simulink library "mylib"  (R2020a)
settings: Solver=VariableStepAuto  StartTime=0.0  StopTime=10.0  RelTol=1e-3
undefined symbols (not defined in the file): d_du_max_pu, dir_to_bus1, dir_to_bus_0L, dir_to_bus_2, dir_to_line1, dir_to_line_0L, dir_to_line_2, du_max_pu, du_ph_max_pu, Fi_0, Fi_T_H, Fi_T_L, Fi_T_M, I0_calc_0L, I0_comp_H, I0_comp_L, I0_comp_M, I0_max_0L, I2_max_2, I_diff1, I_diff2, I_diff3, I_diff4, I_diff5, I_diff_to, I_hight_CT1_G, I_hight_CT2_G, I_low_CT1, I_low_CT2, I_max1, I_max2, I_max3, I_max4, I_max5, I_min_sec_CT1, I_min_sec_CT2, I_unb, Iph_max_0L, Iph_max_2, jmp_in_zone, jmp_in_zone_0L, jmp_in_zone_2, K_dop, max_min1, only_K1_0L, only_K1_2, only_K2_0L, only_K2_2, only_K3_0L, only_K3_2, P_ctl_0, PQ_Fi_ctl_0, Q_ctl_0, S_set_0, set, set1, T_fast, T_I_ctl, T_off, T_on ... (+15)
libraries: $bdroot x184, powerlib_meascontrol x97
(part 7 of 14)

== system mylib/278_dzt_v1/diff_brake/calc_brake_Ia ==
  I_max : Inport
  I_diff_to : Inport  Port=2
  I_diff_1 : Inport  Port=3
  I_max_1 : Inport  Port=4
  I_diff_2 : Inport  Port=5
  I_max_2 : Inport  Port=6
  I_diff_3 : Inport  Port=7
  I_max_3 : Inport  Port=8
  I_diff_4 : Inport  Port=9
  I_max_4 : Inport  Port=10
  I_diff_5 : Inport  Port=11
  I_max_5 : Inport  Port=12
  31 : Constant  Value=0
  cut_brake_1 : Subsystem
  cut_brake_2 : Subsystem
  cut_brake_3 : Subsystem
  cut_brake_4 : Subsystem
  I_brake : Outport
  wires:
  I_diff_5/1 -> cut_brake_3/7(I_diff_next), cut_brake_4/5(I_diff_cur2)
  I_max_5/1 -> cut_brake_3/8(I_max_next), cut_brake_4/6(I_max_cur2)
  cut_brake_3/1(I_brake) -> cut_brake_4/1(Y_in)
  cut_brake_2/1(I_brake) -> cut_brake_3/1(Y_in)
  I_max_4/1 -> cut_brake_3/6(I_max_cur2), cut_brake_4/4(I_max_cur1), cut_brake_2/8(I_max_next)
  I_diff_4/1 -> cut_brake_2/7(I_diff_next), cut_brake_4/3(I_diff_cur1), cut_brake_3/5(I_diff_cur2)
  cut_brake_1/1(I_brake) -> cut_brake_2/1(Y_in)
  31/1 -> cut_brake_1/1(Y_in), cut_brake_4/7(I_diff_next), cut_brake_4/8(I_max_next)
  I_max/1 -> cut_brake_1/2(I_max), cut_brake_2/2(I_max), cut_brake_3/2(I_max), cut_brake_4/2(I_max)
  I_max_3/1 -> cut_brake_1/8(I_max_next), cut_brake_2/6(I_max_cur2), cut_brake_3/4(I_max_cur1)
  I_diff_3/1 -> cut_brake_1/7(I_diff_next), cut_brake_2/5(I_diff_cur2), cut_brake_3/3(I_diff_cur1)
  I_max_2/1 -> cut_brake_1/6(I_max_cur2), cut_brake_2/4(I_max_cur1)
  I_diff_2/1 -> cut_brake_1/5(I_diff_cur2), cut_brake_2/3(I_diff_cur1)
  I_max_1/1 -> cut_brake_1/4(I_max_cur1)
  I_diff_1/1 -> cut_brake_1/3(I_diff_cur1)
  I_diff_to/1 -> cut_brake_1/9(I_diff_to), cut_brake_2/9(I_diff_to), cut_brake_3/9(I_diff_to), cut_brake_4/9(I_diff_to)
  cut_brake_4/1(I_brake) -> I_brake/1

== system mylib/278_dzt_v1/diff_brake/calc_brake_Ib ==
  I_max : Inport
  I_diff_to : Inport  Port=2
  I_diff_1 : Inport  Port=3
  I_max_1 : Inport  Port=4
  I_diff_2 : Inport  Port=5
  I_max_2 : Inport  Port=6
  I_diff_3 : Inport  Port=7
  I_max_3 : Inport  Port=8
  I_diff_4 : Inport  Port=9
  I_max_4 : Inport  Port=10
  I_diff_5 : Inport  Port=11
  I_max_5 : Inport  Port=12
  31 : Constant  Value=0
  cut_brake_1 : Subsystem
  cut_brake_2 : Subsystem
  cut_brake_3 : Subsystem
  cut_brake_4 : Subsystem
  I_brake : Outport
  wires:
  I_diff_5/1 -> cut_brake_3/7(I_diff_next), cut_brake_4/5(I_diff_cur2)
  I_max_5/1 -> cut_brake_3/8(I_max_next), cut_brake_4/6(I_max_cur2)
  cut_brake_3/1(I_brake) -> cut_brake_4/1(Y_in)
  cut_brake_2/1(I_brake) -> cut_brake_3/1(Y_in)
  I_max_4/1 -> cut_brake_3/6(I_max_cur2), cut_brake_4/4(I_max_cur1), cut_brake_2/8(I_max_next)
  I_diff_4/1 -> cut_brake_2/7(I_diff_next), cut_brake_4/3(I_diff_cur1), cut_brake_3/5(I_diff_cur2)
  cut_brake_1/1(I_brake) -> cut_brake_2/1(Y_in)
  31/1 -> cut_brake_1/1(Y_in), cut_brake_4/7(I_diff_next), cut_brake_4/8(I_max_next)
  I_max/1 -> cut_brake_1/2(I_max), cut_brake_2/2(I_max), cut_brake_3/2(I_max), cut_brake_4/2(I_max)
  I_max_3/1 -> cut_brake_1/8(I_max_next), cut_brake_2/6(I_max_cur2), cut_brake_3/4(I_max_cur1)
  I_diff_3/1 -> cut_brake_1/7(I_diff_next), cut_brake_2/5(I_diff_cur2), cut_brake_3/3(I_diff_cur1)
  I_max_2/1 -> cut_brake_1/6(I_max_cur2), cut_brake_2/4(I_max_cur1)
  I_diff_2/1 -> cut_brake_1/5(I_diff_cur2), cut_brake_2/3(I_diff_cur1)
  I_max_1/1 -> cut_brake_1/4(I_max_cur1)
  I_diff_1/1 -> cut_brake_1/3(I_diff_cur1)
  I_diff_to/1 -> cut_brake_1/9(I_diff_to), cut_brake_2/9(I_diff_to), cut_brake_3/9(I_diff_to), cut_brake_4/9(I_diff_to)
  cut_brake_4/1(I_brake) -> I_brake/1

== system mylib/278_dzt_v1/diff_brake/calc_brake_Ic ==
  I_max : Inport
  I_diff_to : Inport  Port=2
  I_diff_1 : Inport  Port=3
  I_max_1 : Inport  Port=4
  I_diff_2 : Inport  Port=5
  I_max_2 : Inport  Port=6
  I_diff_3 : Inport  Port=7
  I_max_3 : Inport  Port=8
  I_diff_4 : Inport  Port=9
  I_max_4 : Inport  Port=10
  I_diff_5 : Inport  Port=11
  I_max_5 : Inport  Port=12
  31 : Constant  Value=0
  cut_brake_1 : Subsystem
  cut_brake_2 : Subsystem
  cut_brake_3 : Subsystem
  cut_brake_4 : Subsystem
  I_brake : Outport
  wires:
  I_diff_5/1 -> cut_brake_3/7(I_diff_next), cut_brake_4/5(I_diff_cur2)
  I_max_5/1 -> cut_brake_3/8(I_max_next), cut_brake_4/6(I_max_cur2)
  cut_brake_3/1(I_brake) -> cut_brake_4/1(Y_in)
  cut_brake_2/1(I_brake) -> cut_brake_3/1(Y_in)
  I_max_4/1 -> cut_brake_3/6(I_max_cur2), cut_brake_4/4(I_max_cur1), cut_brake_2/8(I_max_next)
  I_diff_4/1 -> cut_brake_2/7(I_diff_next), cut_brake_4/3(I_diff_cur1), cut_brake_3/5(I_diff_cur2)
  cut_brake_1/1(I_brake) -> cut_brake_2/1(Y_in)
  31/1 -> cut_brake_1/1(Y_in), cut_brake_4/7(I_diff_next), cut_brake_4/8(I_max_next)
  I_max/1 -> cut_brake_1/2(I_max), cut_brake_2/2(I_max), cut_brake_3/2(I_max), cut_brake_4/2(I_max)
  I_max_3/1 -> cut_brake_1/8(I_max_next), cut_brake_2/6(I_max_cur2), cut_brake_3/4(I_max_cur1)
  I_diff_3/1 -> cut_brake_1/7(I_diff_next), cut_brake_2/5(I_diff_cur2), cut_brake_3/3(I_diff_cur1)
  I_max_2/1 -> cut_brake_1/6(I_max_cur2), cut_brake_2/4(I_max_cur1)
  I_diff_2/1 -> cut_brake_1/5(I_diff_cur2), cut_brake_2/3(I_diff_cur1)
  I_max_1/1 -> cut_brake_1/4(I_max_cur1)
  I_diff_1/1 -> cut_brake_1/3(I_diff_cur1)
  I_diff_to/1 -> cut_brake_1/9(I_diff_to), cut_brake_2/9(I_diff_to), cut_brake_3/9(I_diff_to), cut_brake_4/9(I_diff_to)
  cut_brake_4/1(I_brake) -> I_brake/1

== system mylib/278_dzt_v1/diff_comp18_ph/diff_comp_a ==
  I_diff : Inport
  I_brake : Inport  Port=2
  I_diff_to : Inport  Port=3
  10 : Logic  AllPortsSameDT=off  OutDataTypeStr=boolean
  11 : Logic  Operator=NOT  AllPortsSameDT=off  OutDataTypeStr=boolean
  2 : RelationalOperator  Operator=>  OutDataTypeStr=boolean  RndMeth=Simplest
  25 : Constant  Value=0
  3 : RelationalOperator  Operator=>  OutDataTypeStr=boolean  RndMeth=Simplest
  4 : RelationalOperator  Operator===  OutDataTypeStr=boolean  RndMeth=Simplest
  5 : RelationalOperator  Operator===  OutDataTypeStr=boolean  RndMeth=Simplest
  7 : Logic  Operator=OR  AllPortsSameDT=off  OutDataTypeStr=boolean
  8 : Logic  AllPortsSameDT=off  OutDataTypeStr=boolean
  9 : Logic  Operator=NOT  AllPortsSameDT=off  OutDataTypeStr=boolean
  Y : Outport
  wires:
  7/1 -> Y/1
  10/1 -> 7/2
  8/1 -> 7/1
  5/1 -> 11/1
  4/1 -> 9/1
  3/1 -> 10/1
  2/1 -> 8/1
  9/1 -> 8/2
  11/1 -> 10/2
  25/1 -> 5/2, 4/2
  I_diff_to/1 -> 3/2, 5/1
  I_brake/1 -> 2/2, 4/1
  I_diff/1 -> 2/1, 3/1

== system mylib/278_dzt_v1/diff_comp18_ph/diff_comp_b ==
  I_diff : Inport
  I_brake : Inport  Port=2
  I_diff_to : Inport  Port=3
  10 : Logic  AllPortsSameDT=off  OutDataTypeStr=boolean
  11 : Logic  Operator=NOT  AllPortsSameDT=off  OutDataTypeStr=boolean
  2 : RelationalOperator  Operator=>  OutDataTypeStr=boolean  RndMeth=Simplest
  25 : Constant  Value=0
  3 : RelationalOperator  Operator=>  OutDataTypeStr=boolean  RndMeth=Simplest
  4 : RelationalOperator  Operator===  OutDataTypeStr=boolean  RndMeth=Simplest
  5 : RelationalOperator  Operator===  OutDataTypeStr=boolean  RndMeth=Simplest
  7 : Logic  Operator=OR  AllPortsSameDT=off  OutDataTypeStr=boolean
  8 : Logic  AllPortsSameDT=off  OutDataTypeStr=boolean
  9 : Logic  Operator=NOT  AllPortsSameDT=off  OutDataTypeStr=boolean
  Y : Outport
  wires:
  7/1 -> Y/1
  10/1 -> 7/2
  8/1 -> 7/1
  5/1 -> 11/1
  4/1 -> 9/1
  3/1 -> 10/1
  2/1 -> 8/1
  9/1 -> 8/2
  11/1 -> 10/2
  25/1 -> 5/2, 4/2
  I_diff_to/1 -> 3/2, 5/1
  I_brake/1 -> 2/2, 4/1
  I_diff/1 -> 2/1, 3/1

== system mylib/278_dzt_v1/diff_comp18_ph/diff_comp_c ==
  I_diff : Inport
  I_brake : Inport  Port=2
  I_diff_to : Inport  Port=3
  10 : Logic  AllPortsSameDT=off  OutDataTypeStr=boolean
  11 : Logic  Operator=NOT  AllPortsSameDT=off  OutDataTypeStr=boolean
  2 : RelationalOperator  Operator=>  OutDataTypeStr=boolean  RndMeth=Simplest
  25 : Constant  Value=0
  3 : RelationalOperator  Operator=>  OutDataTypeStr=boolean  RndMeth=Simplest
  4 : RelationalOperator  Operator===  OutDataTypeStr=boolean  RndMeth=Simplest
  5 : RelationalOperator  Operator===  OutDataTypeStr=boolean  RndMeth=Simplest
  7 : Logic  Operator=OR  AllPortsSameDT=off  OutDataTypeStr=boolean
  8 : Logic  AllPortsSameDT=off  OutDataTypeStr=boolean
  9 : Logic  Operator=NOT  AllPortsSameDT=off  OutDataTypeStr=boolean
  Y : Outport
  wires:
  7/1 -> Y/1
  10/1 -> 7/2
  8/1 -> 7/1
  5/1 -> 11/1
  4/1 -> 9/1
  3/1 -> 10/1
  2/1 -> 8/1
  9/1 -> 8/2
  11/1 -> 10/2
  25/1 -> 5/2, 4/2
  I_diff_to/1 -> 3/2, 5/1
  I_brake/1 -> 2/2, 4/1
  I_diff/1 -> 2/1, 3/1

== system mylib/278_dzt_v1/diff_trans_calc_H/Ia_calc ==
  I_re_in : Inport
  I_im_in : Inport  Port=2
  I30_re : Inport  Port=3
  I30_im : Inport  Port=4
  K_CT : Inport  Port=5
  K_T : Inport  Port=6
  I0_comp : Inport  Port=7
  Fi_CT : Inport  Port=8
  Fi_T : Inport  Port=9
  1 : Constant  Value=0.017453292519
  10 : Sum  Inputs=+-
  {2..4,11..13} (6 alike) : Product
  14 : Sum  Inputs=+-
  5 : Sum  Inputs=+-
  6 : Switch  Criteria=u2 > Threshold
  7 : Switch  Criteria=u2 > Threshold
  8 : Trigonometry
  9 : Trigonometry  Operator=cos
  module : $bdroot/module  SystemSampleTime=-1  Latency=0  AutoFrameSizeCalculation=off
  orto_MUL_orto : Subsystem
  orto_to_arg : Subsystem
  I_re : Outport
  I_im : Outport  Port=2
  I_eff : Outport  Port=3
  I_arg : Outport  Port=4
  wires:
  I0_comp/1 -> 7/2, 6/2
  14/1 -> 6/1
  5/1 -> 7/1
  13/1 -> 14/2
  12/1 -> 5/2
  4/1 -> 14/1, 6/3
  3/1 -> 5/1, 7/3
  2/1 -> 3/2, 4/2, 12/2, 13/2
  I30_im/1 -> 13/1
  I30_re/1 -> 12/1
  11/1 -> 9/1, 8/1
  1/1 -> 11/2
  10/1 -> 11/1
  Fi_T/1 -> 10/2
  Fi_CT/1 -> 10/1
  8/1 -> orto_MUL_orto/4(F2im)
  9/1 -> orto_MUL_orto/3(F2re)
  7/1 -> orto_MUL_orto/1(F1re)
  6/1 -> orto_MUL_orto/2(F1im)
  orto_MUL_orto/2(Fim) -> I_im/1, module/2, orto_to_arg/2(im)
  orto_MUL_orto/1(Fre) -> I_re/1, module/1, orto_to_arg/1(re)
  module/1 -> I_eff/1
  orto_to_arg/1(arg) -> I_arg/1
  I_im_in/1 -> 4/1
  I_re_in/1 -> 3/1
  K_T/1 -> 2/2
  K_CT/1 -> 2/1

== system mylib/278_dzt_v1/diff_trans_calc_H/Ia_diff_calc ==
  I_re_1 : Inport
  I_im_1 : Inport  Port=2
  I_re_2 : Inport  Port=3
  I_im_2 : Inport  Port=4
  fix : Inport  Port=5
  I_re_max_in : Inport  Port=6
  I_im_max_in : Inport  Port=7
  in_range_I : Inport  Port=8
  {1,3..6,12} (6 alike) : Switch  Criteria=u2 > Threshold
  10 : RelationalOperator  Operator=>  OutDataTypeStr=boolean  RndMeth=Simplest
  11 : Sum
  154 : Constant  Value=0
  2 : Sum
  module1 : Subsystem
  module2 : Subsystem
  I_re_diff : Outport
  I_im_diff1 : Outport  Port=2
  I_re_max : Outport  Port=3
  I_im_max : Outport  Port=4
  wires:
  fix/1 -> 4/2, 3/2
  I_re_2/1 -> 6/3
  I_im_2/1 -> 5/3
  I_im_max_in/1 -> module1/2(Im), 1/1
  I_re_max_in/1 -> 12/1, module1/1(Re)
  4/1 -> 2/2, 12/3, module2/1(Re)
  3/1 -> 1/3, 11/2, module2/2(Im)
  154/1 -> 5/1, 6/1, 4/3, 3/3
  in_range_I/1 -> 5/2, 6/2
  5/1 -> 3/1
  6/1 -> 4/1
  module2/1(Module) -> 10/2
  module1/1(Module) -> 10/1
  I_im_1/1 -> 11/1
  I_re_1/1 -> 2/1
  10/1 -> 1/2, 12/2
  2/1 -> I_re_diff/1
  11/1 -> I_im_diff1/1
  1/1 -> I_im_max/1
  12/1 -> I_re_max/1

== system mylib/278_dzt_v1/diff_trans_calc_H/Ib_calc ==
  I_re_in : Inport
  I_im_in : Inport  Port=2
  I30_re : Inport  Port=3
  I30_im : Inport  Port=4
  K_CT : Inport  Port=5
  K_T : Inport  Port=6
  I0_comp : Inport  Port=7
  Fi_CT : Inport  Port=8
  Fi_T : Inport  Port=9
  1 : Constant  Value=0.017453292519
  10 : Sum  Inputs=+-
  {2..4,11..13} (6 alike) : Product
  14 : Sum  Inputs=+-
  5 : Sum  Inputs=+-
  6 : Switch  Criteria=u2 > Threshold
  7 : Switch  Criteria=u2 > Threshold
  8 : Trigonometry
  9 : Trigonometry  Operator=cos
  module : $bdroot/module  SystemSampleTime=-1  Latency=0  AutoFrameSizeCalculation=off
  orto_MUL_orto : Subsystem
  orto_to_arg : Subsystem
  I_re : Outport
  I_im : Outport  Port=2
  I_eff : Outport  Port=3
  I_arg : Outport  Port=4
  wires:
  I0_comp/1 -> 7/2, 6/2
  14/1 -> 6/1
  5/1 -> 7/1
  13/1 -> 14/2
  12/1 -> 5/2
  4/1 -> 14/1, 6/3
  3/1 -> 5/1, 7/3
  2/1 -> 3/2, 4/2, 12/2, 13/2
  I30_im/1 -> 13/1
  I30_re/1 -> 12/1
  11/1 -> 9/1, 8/1
  1/1 -> 11/2
  10/1 -> 11/1
  Fi_T/1 -> 10/2
  Fi_CT/1 -> 10/1
  8/1 -> orto_MUL_orto/4(F2im)
  9/1 -> orto_MUL_orto/3(F2re)
  7/1 -> orto_MUL_orto/1(F1re)
  6/1 -> orto_MUL_orto/2(F1im)
  orto_MUL_orto/2(Fim) -> I_im/1, module/2, orto_to_arg/2(im)
  orto_MUL_orto/1(Fre) -> I_re/1, module/1, orto_to_arg/1(re)
  module/1 -> I_eff/1
  orto_to_arg/1(arg) -> I_arg/1
  I_im_in/1 -> 4/1
  I_re_in/1 -> 3/1
  K_T/1 -> 2/2
  K_CT/1 -> 2/1

== system mylib/278_dzt_v1/diff_trans_calc_H/Ib_diff_calc ==
  I_re_1 : Inport
  I_im_1 : Inport  Port=2
  I_re_2 : Inport  Port=3
  I_im_2 : Inport  Port=4
  fix : Inport  Port=5
  I_re_max_in : Inport  Port=6
  I_im_max_in : Inport  Port=7
  in_range_I : Inport  Port=8
  {1,3..6,12} (6 alike) : Switch  Criteria=u2 > Threshold
  10 : RelationalOperator  Operator=>  OutDataTypeStr=boolean  RndMeth=Simplest
  11 : Sum
  154 : Constant  Value=0
  2 : Sum
  module1 : Subsystem
  module2 : Subsystem
  I_re_diff : Outport
  I_im_diff1 : Outport  Port=2
  I_re_max : Outport  Port=3
  I_im_max : Outport  Port=4
  wires:
  fix/1 -> 4/2, 3/2
  I_re_2/1 -> 6/3
  I_im_2/1 -> 5/3
  I_im_max_in/1 -> module1/2(Im), 1/1
  I_re_max_in/1 -> 12/1, module1/1(Re)
  4/1 -> 2/2, 12/3, module2/1(Re)
  3/1 -> 1/3, 11/2, module2/2(Im)
  154/1 -> 5/1, 6/1, 4/3, 3/3
  in_range_I/1 -> 5/2, 6/2
  5/1 -> 3/1
  6/1 -> 4/1
  module2/1(Module) -> 10/2
  module1/1(Module) -> 10/1
  I_im_1/1 -> 11/1
  I_re_1/1 -> 2/1
  10/1 -> 1/2, 12/2
  2/1 -> I_re_diff/1
  11/1 -> I_im_diff1/1
  1/1 -> I_im_max/1
  12/1 -> I_re_max/1

== system mylib/278_dzt_v1/diff_trans_calc_H/Ic_calc ==
  I_re_in : Inport
  I_im_in : Inport  Port=2
  I30_re : Inport  Port=3
  I30_im : Inport  Port=4
  K_CT : Inport  Port=5
  K_T : Inport  Port=6
  I0_comp : Inport  Port=7
  Fi_CT : Inport  Port=8
  Fi_T : Inport  Port=9
  1 : Constant  Value=0.017453292519
  10 : Sum  Inputs=+-
  {2..4,11..13} (6 alike) : Product
  14 : Sum  Inputs=+-
  5 : Sum  Inputs=+-
  6 : Switch  Criteria=u2 > Threshold
  7 : Switch  Criteria=u2 > Threshold
  8 : Trigonometry
  9 : Trigonometry  Operator=cos
  module : $bdroot/module  SystemSampleTime=-1  Latency=0  AutoFrameSizeCalculation=off
  orto_MUL_orto : Subsystem
  orto_to_arg : Subsystem
  I_re : Outport
  I_im : Outport  Port=2
  I_eff : Outport  Port=3
  I_arg : Outport  Port=4
  wires:
  I0_comp/1 -> 7/2, 6/2
  14/1 -> 6/1
  5/1 -> 7/1
  13/1 -> 14/2
  12/1 -> 5/2
  4/1 -> 14/1, 6/3
  3/1 -> 5/1, 7/3
  2/1 -> 3/2, 4/2, 12/2, 13/2
  I30_im/1 -> 13/1
  I30_re/1 -> 12/1
  11/1 -> 9/1, 8/1
  1/1 -> 11/2
  10/1 -> 11/1
  Fi_T/1 -> 10/2
  Fi_CT/1 -> 10/1
  8/1 -> orto_MUL_orto/4(F2im)
  9/1 -> orto_MUL_orto/3(F2re)
  7/1 -> orto_MUL_orto/1(F1re)
  6/1 -> orto_MUL_orto/2(F1im)
  orto_MUL_orto/2(Fim) -> I_im/1, module/2, orto_to_arg/2(im)
  orto_MUL_orto/1(Fre) -> I_re/1, module/1, orto_to_arg/1(re)
  module/1 -> I_eff/1
  orto_to_arg/1(arg) -> I_arg/1
  I_im_in/1 -> 4/1
  I_re_in/1 -> 3/1
  K_T/1 -> 2/2
  K_CT/1 -> 2/1

== system mylib/278_dzt_v1/diff_trans_calc_H/Ic_diff_calc ==
  I_re_1 : Inport
  I_im_1 : Inport  Port=2
  I_re_2 : Inport  Port=3
  I_im_2 : Inport  Port=4
  fix : Inport  Port=5
  I_re_max_in : Inport  Port=6
  I_im_max_in : Inport  Port=7
  in_range_I : Inport  Port=8
  {1,3..6,12} (6 alike) : Switch  Criteria=u2 > Threshold
  10 : RelationalOperator  Operator=>  OutDataTypeStr=boolean  RndMeth=Simplest
  11 : Sum
  154 : Constant  Value=0
  2 : Sum
  module1 : Subsystem
  module2 : Subsystem
  I_re_diff : Outport
  I_im_diff1 : Outport  Port=2
  I_re_max : Outport  Port=3
  I_im_max : Outport  Port=4
  wires:
  fix/1 -> 4/2, 3/2
  I_re_2/1 -> 6/3
  I_im_2/1 -> 5/3
  I_im_max_in/1 -> module1/2(Im), 1/1
  I_re_max_in/1 -> 12/1, module1/1(Re)
  4/1 -> 2/2, 12/3, module2/1(Re)
  3/1 -> 1/3, 11/2, module2/2(Im)
  154/1 -> 5/1, 6/1, 4/3, 3/3
  in_range_I/1 -> 5/2, 6/2
  5/1 -> 3/1
  6/1 -> 4/1
  module2/1(Module) -> 10/2
  module1/1(Module) -> 10/1
  I_im_1/1 -> 11/1
  I_re_1/1 -> 2/1
  10/1 -> 1/2, 12/2
  2/1 -> I_re_diff/1
  11/1 -> I_im_diff1/1
  1/1 -> I_im_max/1
  12/1 -> I_re_max/1

== system mylib/278_dzt_v1/diff_trans_calc_H/jmp_cnt18_ph ==
  cnt_jmp0_in : Inport
  cnt_jmp_in : Inport  Port=2
  Ia_zero_in : Inport  Port=3
  Ib_zero_in : Inport  Port=4
  Ic_zero_in : Inport  Port=5
  Iall_zero_in : Inport  Port=6
  in_range_Ia : Inport  Port=7
  in_range_Ib : Inport  Port=8
  in_range_Ic : Inport  Port=9
  jmp_Ia : Inport  Port=10
  jmp_Ib : Inport  Port=11
  jmp_Ic : Inport  Port=12
  fix : Inport  Port=13
  {1,3,5..7,10} (6 alike) : Logic  AllPortsSameDT=off  OutDataTypeStr=boolean
  11 : Logic  Operator=NOT  AllPortsSameDT=off  OutDataTypeStr=boolean
  12 : Logic  Operator=OR  AllPortsSameDT=off  OutDataTypeStr=boolean
  13 : Logic  Operator=OR  AllPortsSameDT=off  OutDataTypeStr=boolean
  14 : Logic  Operator=OR  AllPortsSameDT=off  OutDataTypeStr=boolean
  15 : Logic  Inputs=4  AllPortsSameDT=off  OutDataTypeStr=boolean
  16 : Switch  Criteria=u2 > Threshold
  17 : Switch  Criteria=u2 > Threshold
  18 : Sum
  19 : Constant
  2 : Logic  Operator=NOT  AllPortsSameDT=off  OutDataTypeStr=boolean
  20 : Sum
  21 : Constant
  4 : Logic  Operator=NOT  AllPortsSameDT=off  OutDataTypeStr=boolean
  8 : Logic  Operator=OR  Inputs=3  AllPortsSameDT=off  OutDataTypeStr=boolean
  9 : Logic  Operator=OR  Inputs=3  AllPortsSameDT=off  OutDataTypeStr=boolean
  R_TRIG : $bdroot/R_TRIG  SystemSampleTime=-1  Latency=0  AutoFrameSizeCalculation=off
  R_TRIG1 : $bdroot/R_TRIG  SystemSampleTime=-1  Latency=0  AutoFrameSizeCalculation=off
  R_TRIG2 : $bdroot/R_TRIG  SystemSampleTime=-1  Latency=0  AutoFrameSizeCalculation=off
  cnt_jmp0 : Outport
  cnt_jmp : Outport  Port=2
  Ia_zero : Outport  Port=3
  Ib_zero : Outport  Port=4
  Ic_zero : Outport  Port=5
  Iall_zero : Outport  Port=6
  wires:
  cnt_jmp0_in/1 -> 16/3, 20/1
  R_TRIG2/1 -> 9/3, 6/2
  fix/1 -> 10/2, 1/2, 3/2
  cnt_jmp_in/1 -> 17/3, 18/1
  9/1 -> 17/2
  20/1 -> 16/1
  21/1 -> 20/2
  19/1 -> 18/2
  18/1 -> 17/1
  17/1 -> cnt_jmp/1
  16/1 -> cnt_jmp0/1
  8/1 -> 16/2
  15/1 -> Iall_zero/1
  14/1 -> Ic_zero/1
  13/1 -> Ib_zero/1
  12/1 -> Ia_zero/1
  Ia_zero_in/1 -> 12/1
  Ib_zero_in/1 -> 13/1
  Ic_zero_in/1 -> 14/1
  Iall_zero_in/1 -> 15/1
  R_TRIG1/1 -> 9/2, 5/2
  R_TRIG/1 -> 9/1, 7/2
  6/1 -> 8/3
  7/1 -> 8/1
  5/1 -> 8/2
  10/1 -> 6/1, 15/4, 14/2
  1/1 -> 5/1, 15/3, 13/2
  3/1 -> 7/1, 15/2, 12/2
  in_range_Ia/1 -> 4/1
  4/1 -> 3/1
  in_range_Ib/1 -> 2/1
  2/1 -> 1/1
  in_range_Ic/1 -> 11/1
  11/1 -> 10/1
  jmp_Ib/1 -> R_TRIG1/1
  jmp_Ic/1 -> R_TRIG2/1
  jmp_Ia/1 -> R_TRIG/1

== system mylib/278_dzt_v1/diff_trans_calc_H/simpcomp ==
  FAre : Inport
  FAim : Inport  Port=2
  FBre : Inport  Port=3
  FBim : Inport  Port=4
  FCre : Inport  Port=5
  FCim : Inport  Port=6
  1 : Constant  Value=-0.5
  {3..5,9..11,18..23} (12 alike) : Sum
  {2,12..16} (6 alike) : Product
  17 : Constant  Value=0.33333333333
  6 : Constant  Value=0.8660254037844386
  7 : Constant  Value=-0.8660254037844386
  orto_MUL_orto : Subsystem
  orto_MUL_orto1 : Subsystem
  orto_MUL_orto2 : Subsystem
  orto_MUL_orto3 : Subsystem
  F0re : Outport
  F0im : Outport  Port=2
  F1re : Outport  Port=3
  F1im : Outport  Port=4
  F2re : Outport  Port=5
  F2im : Outport  Port=6
  wires:
  1/1 -> orto_MUL_orto1/3(F2re), orto_MUL_orto/3(F2re), orto_MUL_orto2/3(F2re), orto_MUL_orto3/3(F2re)
  6/1 -> orto_MUL_orto2/4(F2im), orto_MUL_orto/4(F2im)
  7/1 -> orto_MUL_orto3/4(F2im), orto_MUL_orto1/4(F2im)
  15/1 -> F2im/1
  14/1 -> F2re/1
  16/1 -> F1im/1
  13/1 -> F1re/1
  2/1 -> F0re/1
  12/1 -> F0im/1
  5/1 -> 2/1
  3/1 -> 12/1
  4/1 -> 13/1
  11/1 -> 16/1
  9/1 -> 14/1
  10/1 -> 15/1
  20/1 -> 10/2
  23/1 -> 9/2
  21/1 -> 11/2
  22/1 -> 4/2
  18/1 -> 3/1
  19/1 -> 5/1
  FAim/1 -> 10/1, 3/2, 11/1
  FAre/1 -> 9/1, 5/2, 4/1
  orto_MUL_orto2/2(Fim) -> 20/2
  orto_MUL_orto1/2(Fim) -> 20/1
  orto_MUL_orto2/1(Fre) -> 23/2
  orto_MUL_orto1/1(Fre) -> 23/1
  orto_MUL_orto3/2(Fim) -> 21/2
  orto_MUL_orto/2(Fim) -> 21/1
  orto_MUL_orto3/1(Fre) -> 22/2
  orto_MUL_orto/1(Fre) -> 22/1
  FBre/1 -> orto_MUL_orto1/1(F1re), 19/1, orto_MUL_orto/1(F1re)
  FBim/1 -> orto_MUL_orto1/2(F1im), 18/1, orto_MUL_orto/2(F1im)
  FCim/1 -> 18/2, orto_MUL_orto2/2(F1im), orto_MUL_orto3/2(F1im)
  FCre/1 -> orto_MUL_orto3/1(F1re), 19/2, orto_MUL_orto2/1(F1re)
  17/1 -> 15/2, 14/2, 13/2, 12/2, 2/2, 16/2

== system mylib/278_dzt_v1/diff_trans_calc_H1/Ia_calc ==
  I_re_in : Inport
  I_im_in : Inport  Port=2
  I30_re : Inport  Port=3
  I30_im : Inport  Port=4
  K_CT : Inport  Port=5
  K_T : Inport  Port=6
  I0_comp : Inport  Port=7
  Fi_CT : Inport  Port=8
  Fi_T : Inport  Port=9
  1 : Constant  Value=0.017453292519
  10 : Sum  Inputs=+-
  {2..4,11..13} (6 alike) : Product
  14 : Sum  Inputs=+-
  5 : Sum  Inputs=+-
  6 : Switch  Criteria=u2 > Threshold
  7 : Switch  Criteria=u2 > Threshold
  8 : Trigonometry
  9 : Trigonometry  Operator=cos
  module : $bdroot/module  SystemSampleTime=-1  Latency=0  AutoFrameSizeCalculation=off
  orto_MUL_orto : Subsystem
  orto_to_arg : Subsystem
  I_re : Outport
  I_im : Outport  Port=2
  I_eff : Outport  Port=3
  I_arg : Outport  Port=4
  wires:
  I0_comp/1 -> 7/2, 6/2
  14/1 -> 6/1
  5/1 -> 7/1
  13/1 -> 14/2
  12/1 -> 5/2
  4/1 -> 14/1, 6/3
  3/1 -> 5/1, 7/3
  2/1 -> 3/2, 4/2, 12/2, 13/2
  I30_im/1 -> 13/1
  I30_re/1 -> 12/1
  11/1 -> 9/1, 8/1
  1/1 -> 11/2
  10/1 -> 11/1
  Fi_T/1 -> 10/2
  Fi_CT/1 -> 10/1
  8/1 -> orto_MUL_orto/4(F2im)
  9/1 -> orto_MUL_orto/3(F2re)
  7/1 -> orto_MUL_orto/1(F1re)
  6/1 -> orto_MUL_orto/2(F1im)
  orto_MUL_orto/2(Fim) -> I_im/1, module/2, orto_to_arg/2(im)
  orto_MUL_orto/1(Fre) -> I_re/1, module/1, orto_to_arg/1(re)
  module/1 -> I_eff/1
  orto_to_arg/1(arg) -> I_arg/1
  I_im_in/1 -> 4/1
  I_re_in/1 -> 3/1
  K_T/1 -> 2/2
  K_CT/1 -> 2/1

== system mylib/278_dzt_v1/diff_trans_calc_H1/Ia_diff_calc ==
  I_re_1 : Inport
  I_im_1 : Inport  Port=2
  I_re_2 : Inport  Port=3
  I_im_2 : Inport  Port=4
  fix : Inport  Port=5
  I_re_max_in : Inport  Port=6
  I_im_max_in : Inport  Port=7
  in_range_I : Inport  Port=8
  {1,3..6,12} (6 alike) : Switch  Criteria=u2 > Threshold
  10 : RelationalOperator  Operator=>  OutDataTypeStr=boolean  RndMeth=Simplest
  11 : Sum
  154 : Constant  Value=0
  2 : Sum
  module1 : Subsystem
  module2 : Subsystem
  I_re_diff : Outport
  I_im_diff1 : Outport  Port=2
  I_re_max : Outport  Port=3
  I_im_max : Outport  Port=4
  wires:
  fix/1 -> 4/2, 3/2
  I_re_2/1 -> 6/3
  I_im_2/1 -> 5/3
  I_im_max_in/1 -> module1/2(Im), 1/1
  I_re_max_in/1 -> 12/1, module1/1(Re)
  4/1 -> 2/2, 12/3, module2/1(Re)
  3/1 -> 1/3, 11/2, module2/2(Im)
  154/1 -> 5/1, 6/1, 4/3, 3/3
  in_range_I/1 -> 5/2, 6/2
  5/1 -> 3/1
  6/1 -> 4/1
  module2/1(Module) -> 10/2
  module1/1(Module) -> 10/1
  I_im_1/1 -> 11/1
  I_re_1/1 -> 2/1
  10/1 -> 1/2, 12/2
  2/1 -> I_re_diff/1
  11/1 -> I_im_diff1/1
  1/1 -> I_im_max/1
  12/1 -> I_re_max/1

== system mylib/278_dzt_v1/diff_trans_calc_H1/Ib_calc ==
  I_re_in : Inport
  I_im_in : Inport  Port=2
  I30_re : Inport  Port=3
  I30_im : Inport  Port=4
  K_CT : Inport  Port=5
  K_T : Inport  Port=6
  I0_comp : Inport  Port=7
  Fi_CT : Inport  Port=8
  Fi_T : Inport  Port=9
  1 : Constant  Value=0.017453292519
  10 : Sum  Inputs=+-
  {2..4,11..13} (6 alike) : Product
  14 : Sum  Inputs=+-
  5 : Sum  Inputs=+-
  6 : Switch  Criteria=u2 > Threshold
  7 : Switch  Criteria=u2 > Threshold
  8 : Trigonometry
  9 : Trigonometry  Operator=cos
  module : $bdroot/module  SystemSampleTime=-1  Latency=0  AutoFrameSizeCalculation=off
  orto_MUL_orto : Subsystem
  orto_to_arg : Subsystem
  I_re : Outport
  I_im : Outport  Port=2
  I_eff : Outport  Port=3
  I_arg : Outport  Port=4
  wires:
  I0_comp/1 -> 7/2, 6/2
  14/1 -> 6/1
  5/1 -> 7/1
  13/1 -> 14/2
  12/1 -> 5/2
  4/1 -> 14/1, 6/3
  3/1 -> 5/1, 7/3
  2/1 -> 3/2, 4/2, 12/2, 13/2
  I30_im/1 -> 13/1
  I30_re/1 -> 12/1
  11/1 -> 9/1, 8/1
  1/1 -> 11/2
  10/1 -> 11/1
  Fi_T/1 -> 10/2
  Fi_CT/1 -> 10/1
  8/1 -> orto_MUL_orto/4(F2im)
  9/1 -> orto_MUL_orto/3(F2re)
  7/1 -> orto_MUL_orto/1(F1re)
  6/1 -> orto_MUL_orto/2(F1im)
  orto_MUL_orto/2(Fim) -> I_im/1, module/2, orto_to_arg/2(im)
  orto_MUL_orto/1(Fre) -> I_re/1, module/1, orto_to_arg/1(re)
  module/1 -> I_eff/1
  orto_to_arg/1(arg) -> I_arg/1
  I_im_in/1 -> 4/1
  I_re_in/1 -> 3/1
  K_T/1 -> 2/2
  K_CT/1 -> 2/1

== system mylib/278_dzt_v1/diff_trans_calc_H1/Ib_diff_calc ==
  I_re_1 : Inport
  I_im_1 : Inport  Port=2
  I_re_2 : Inport  Port=3
  I_im_2 : Inport  Port=4
  fix : Inport  Port=5
  I_re_max_in : Inport  Port=6
  I_im_max_in : Inport  Port=7
  in_range_I : Inport  Port=8
  {1,3..6,12} (6 alike) : Switch  Criteria=u2 > Threshold
  10 : RelationalOperator  Operator=>  OutDataTypeStr=boolean  RndMeth=Simplest
  11 : Sum
  154 : Constant  Value=0
  2 : Sum
  module1 : Subsystem
  module2 : Subsystem
  I_re_diff : Outport
  I_im_diff1 : Outport  Port=2
  I_re_max : Outport  Port=3
  I_im_max : Outport  Port=4
  wires:
  fix/1 -> 4/2, 3/2
  I_re_2/1 -> 6/3
  I_im_2/1 -> 5/3
  I_im_max_in/1 -> module1/2(Im), 1/1
  I_re_max_in/1 -> 12/1, module1/1(Re)
  4/1 -> 2/2, 12/3, module2/1(Re)
  3/1 -> 1/3, 11/2, module2/2(Im)
  154/1 -> 5/1, 6/1, 4/3, 3/3
  in_range_I/1 -> 5/2, 6/2
  5/1 -> 3/1
  6/1 -> 4/1
  module2/1(Module) -> 10/2
  module1/1(Module) -> 10/1
  I_im_1/1 -> 11/1
  I_re_1/1 -> 2/1
  10/1 -> 1/2, 12/2
  2/1 -> I_re_diff/1
  11/1 -> I_im_diff1/1
  1/1 -> I_im_max/1
  12/1 -> I_re_max/1

== system mylib/278_dzt_v1/diff_trans_calc_H1/Ic_calc ==
  I_re_in : Inport
  I_im_in : Inport  Port=2
  I30_re : Inport  Port=3
  I30_im : Inport  Port=4
  K_CT : Inport  Port=5
  K_T : Inport  Port=6
  I0_comp : Inport  Port=7
  Fi_CT : Inport  Port=8
  Fi_T : Inport  Port=9
  1 : Constant  Value=0.017453292519
  10 : Sum  Inputs=+-
  {2..4,11..13} (6 alike) : Product
  14 : Sum  Inputs=+-
  5 : Sum  Inputs=+-
  6 : Switch  Criteria=u2 > Threshold
  7 : Switch  Criteria=u2 > Threshold
  8 : Trigonometry
  9 : Trigonometry  Operator=cos
  module : $bdroot/module  SystemSampleTime=-1  Latency=0  AutoFrameSizeCalculation=off
  orto_MUL_orto : Subsystem
  orto_to_arg : Subsystem
  I_re : Outport
  I_im : Outport  Port=2
  I_eff : Outport  Port=3
  I_arg : Outport  Port=4
  wires:
  I0_comp/1 -> 7/2, 6/2
  14/1 -> 6/1
  5/1 -> 7/1
  13/1 -> 14/2
  12/1 -> 5/2
  4/1 -> 14/1, 6/3
  3/1 -> 5/1, 7/3
  2/1 -> 3/2, 4/2, 12/2, 13/2
  I30_im/1 -> 13/1
  I30_re/1 -> 12/1
  11/1 -> 9/1, 8/1
  1/1 -> 11/2
  10/1 -> 11/1
  Fi_T/1 -> 10/2
  Fi_CT/1 -> 10/1
  8/1 -> orto_MUL_orto/4(F2im)
  9/1 -> orto_MUL_orto/3(F2re)
  7/1 -> orto_MUL_orto/1(F1re)
  6/1 -> orto_MUL_orto/2(F1im)
  orto_MUL_orto/2(Fim) -> I_im/1, module/2, orto_to_arg/2(im)
  orto_MUL_orto/1(Fre) -> I_re/1, module/1, orto_to_arg/1(re)
  module/1 -> I_eff/1
  orto_to_arg/1(arg) -> I_arg/1
  I_im_in/1 -> 4/1
  I_re_in/1 -> 3/1
  K_T/1 -> 2/2
  K_CT/1 -> 2/1

== system mylib/278_dzt_v1/diff_trans_calc_H1/Ic_diff_calc ==
  I_re_1 : Inport
  I_im_1 : Inport  Port=2
  I_re_2 : Inport  Port=3
  I_im_2 : Inport  Port=4
  fix : Inport  Port=5
  I_re_max_in : Inport  Port=6
  I_im_max_in : Inport  Port=7
  in_range_I : Inport  Port=8
  {1,3..6,12} (6 alike) : Switch  Criteria=u2 > Threshold
  10 : RelationalOperator  Operator=>  OutDataTypeStr=boolean  RndMeth=Simplest
  11 : Sum
  154 : Constant  Value=0
  2 : Sum
  module1 : Subsystem
  module2 : Subsystem
  I_re_diff : Outport
  I_im_diff1 : Outport  Port=2
  I_re_max : Outport  Port=3
  I_im_max : Outport  Port=4
  wires:
  fix/1 -> 4/2, 3/2
  I_re_2/1 -> 6/3
  I_im_2/1 -> 5/3
  I_im_max_in/1 -> module1/2(Im), 1/1
  I_re_max_in/1 -> 12/1, module1/1(Re)
  4/1 -> 2/2, 12/3, module2/1(Re)
  3/1 -> 1/3, 11/2, module2/2(Im)
  154/1 -> 5/1, 6/1, 4/3, 3/3
  in_range_I/1 -> 5/2, 6/2
  5/1 -> 3/1
  6/1 -> 4/1
  module2/1(Module) -> 10/2
  module1/1(Module) -> 10/1
  I_im_1/1 -> 11/1
  I_re_1/1 -> 2/1
  10/1 -> 1/2, 12/2
  2/1 -> I_re_diff/1
  11/1 -> I_im_diff1/1
  1/1 -> I_im_max/1
  12/1 -> I_re_max/1

== system mylib/278_dzt_v1/diff_trans_calc_H1/jmp_cnt18_ph ==
  cnt_jmp0_in : Inport
  cnt_jmp_in : Inport  Port=2
  Ia_zero_in : Inport  Port=3
  Ib_zero_in : Inport  Port=4
  Ic_zero_in : Inport  Port=5
  Iall_zero_in : Inport  Port=6
  in_range_Ia : Inport  Port=7
  in_range_Ib : Inport  Port=8
  in_range_Ic : Inport  Port=9
  jmp_Ia : Inport  Port=10
  jmp_Ib : Inport  Port=11
  jmp_Ic : Inport  Port=12
  fix : Inport  Port=13
  {1,3,5..7,10} (6 alike) : Logic  AllPortsSameDT=off  OutDataTypeStr=boolean
  11 : Logic  Operator=NOT  AllPortsSameDT=off  OutDataTypeStr=boolean
  12 : Logic  Operator=OR  AllPortsSameDT=off  OutDataTypeStr=boolean
  13 : Logic  Operator=OR  AllPortsSameDT=off  OutDataTypeStr=boolean
  14 : Logic  Operator=OR  AllPortsSameDT=off  OutDataTypeStr=boolean
  15 : Logic  Inputs=4  AllPortsSameDT=off  OutDataTypeStr=boolean
  16 : Switch  Criteria=u2 > Threshold
  17 : Switch  Criteria=u2 > Threshold
  18 : Sum
  19 : Constant
  2 : Logic  Operator=NOT  AllPortsSameDT=off  OutDataTypeStr=boolean
  20 : Sum
  21 : Constant
  4 : Logic  Operator=NOT  AllPortsSameDT=off  OutDataTypeStr=boolean
  8 : Logic  Operator=OR  Inputs=3  AllPortsSameDT=off  OutDataTypeStr=boolean
  9 : Logic  Operator=OR  Inputs=3  AllPortsSameDT=off  OutDataTypeStr=boolean
  R_TRIG : $bdroot/R_TRIG  SystemSampleTime=-1  Latency=0  AutoFrameSizeCalculation=off
  R_TRIG1 : $bdroot/R_TRIG  SystemSampleTime=-1  Latency=0  AutoFrameSizeCalculation=off
  R_TRIG2 : $bdroot/R_TRIG  SystemSampleTime=-1  Latency=0  AutoFrameSizeCalculation=off
  cnt_jmp0 : Outport
  cnt_jmp : Outport  Port=2
  Ia_zero : Outport  Port=3
  Ib_zero : Outport  Port=4
  Ic_zero : Outport  Port=5
  Iall_zero : Outport  Port=6
  wires:
  cnt_jmp0_in/1 -> 16/3, 20/1
  R_TRIG2/1 -> 9/3, 6/2
  fix/1 -> 10/2, 1/2, 3/2
  cnt_jmp_in/1 -> 17/3, 18/1
  9/1 -> 17/2
  20/1 -> 16/1
  21/1 -> 20/2
  19/1 -> 18/2
  18/1 -> 17/1
  17/1 -> cnt_jmp/1
  16/1 -> cnt_jmp0/1
  8/1 -> 16/2
  15/1 -> Iall_zero/1
  14/1 -> Ic_zero/1
  13/1 -> Ib_zero/1
  12/1 -> Ia_zero/1
  Ia_zero_in/1 -> 12/1
  Ib_zero_in/1 -> 13/1
  Ic_zero_in/1 -> 14/1
  Iall_zero_in/1 -> 15/1
  R_TRIG1/1 -> 9/2, 5/2
  R_TRIG/1 -> 9/1, 7/2
  6/1 -> 8/3
  7/1 -> 8/1
  5/1 -> 8/2
  10/1 -> 6/1, 15/4, 14/2
  1/1 -> 5/1, 15/3, 13/2
  3/1 -> 7/1, 15/2, 12/2
  in_range_Ia/1 -> 4/1
  4/1 -> 3/1
  in_range_Ib/1 -> 2/1
  2/1 -> 1/1
  in_range_Ic/1 -> 11/1
  11/1 -> 10/1
  jmp_Ib/1 -> R_TRIG1/1
  jmp_Ic/1 -> R_TRIG2/1
  jmp_Ia/1 -> R_TRIG/1

== system mylib/278_dzt_v1/diff_trans_calc_H1/simpcomp ==
  FAre : Inport
  FAim : Inport  Port=2
  FBre : Inport  Port=3
  FBim : Inport  Port=4
  FCre : Inport  Port=5
  FCim : Inport  Port=6
  1 : Constant  Value=-0.5
  {3..5,9..11,18..23} (12 alike) : Sum
  {2,12..16} (6 alike) : Product
  17 : Constant  Value=0.33333333333
  6 : Constant  Value=0.8660254037844386
  7 : Constant  Value=-0.8660254037844386
  orto_MUL_orto : Subsystem
  orto_MUL_orto1 : Subsystem
  orto_MUL_orto2 : Subsystem
  orto_MUL_orto3 : Subsystem
  F0re : Outport
  F0im : Outport  Port=2
  F1re : Outport  Port=3
  F1im : Outport  Port=4
  F2re : Outport  Port=5
  F2im : Outport  Port=6
  wires:
  1/1 -> orto_MUL_orto1/3(F2re), orto_MUL_orto/3(F2re), orto_MUL_orto2/3(F2re), orto_MUL_orto3/3(F2re)
  6/1 -> orto_MUL_orto2/4(F2im), orto_MUL_orto/4(F2im)
  7/1 -> orto_MUL_orto3/4(F2im), orto_MUL_orto1/4(F2im)
  15/1 -> F2im/1
  14/1 -> F2re/1
  16/1 -> F1im/1
  13/1 -> F1re/1
  2/1 -> F0re/1
  12/1 -> F0im/1
  5/1 -> 2/1
  3/1 -> 12/1
  4/1 -> 13/1
  11/1 -> 16/1
  9/1 -> 14/1
  10/1 -> 15/1
  20/1 -> 10/2
  23/1 -> 9/2
  21/1 -> 11/2
  22/1 -> 4/2
  18/1 -> 3/1
  19/1 -> 5/1
  FAim/1 -> 10/1, 3/2, 11/1
  FAre/1 -> 9/1, 5/2, 4/1
  orto_MUL_orto2/2(Fim) -> 20/2
  orto_MUL_orto1/2(Fim) -> 20/1
  orto_MUL_orto2/1(Fre) -> 23/2
  orto_MUL_orto1/1(Fre) -> 23/1
  orto_MUL_orto3/2(Fim) -> 21/2
  orto_MUL_orto/2(Fim) -> 21/1
  orto_MUL_orto3/1(Fre) -> 22/2
  orto_MUL_orto/1(Fre) -> 22/1
  FBre/1 -> orto_MUL_orto1/1(F1re), 19/1, orto_MUL_orto/1(F1re)
  FBim/1 -> orto_MUL_orto1/2(F1im), 18/1, orto_MUL_orto/2(F1im)
  FCim/1 -> 18/2, orto_MUL_orto2/2(F1im), orto_MUL_orto3/2(F1im)
  FCre/1 -> orto_MUL_orto3/1(F1re), 19/2, orto_MUL_orto2/1(F1re)
  17/1 -> 15/2, 14/2, 13/2, 12/2, 2/2, 16/2

== system mylib/278_dzt_v1/diff_trans_calc_H2/Ia_calc ==
  I_re_in : Inport
  I_im_in : Inport  Port=2
  I30_re : Inport  Port=3
  I30_im : Inport  Port=4
  K_CT : Inport  Port=5
  K_T : Inport  Port=6
  I0_comp : Inport  Port=7
  Fi_CT : Inport  Port=8
  Fi_T : Inport  Port=9
  1 : Constant  Value=0.017453292519
  10 : Sum  Inputs=+-
  {2..4,11..13} (6 alike) : Product
  14 : Sum  Inputs=+-
  5 : Sum  Inputs=+-
  6 : Switch  Criteria=u2 > Threshold
  7 : Switch  Criteria=u2 > Threshold
  8 : Trigonometry
  9 : Trigonometry  Operator=cos
  module : $bdroot/module  SystemSampleTime=-1  Latency=0  AutoFrameSizeCalculation=off
  orto_MUL_orto : Subsystem
  orto_to_arg : Subsystem
  I_re : Outport
  I_im : Outport  Port=2
  I_eff : Outport  Port=3
  I_arg : Outport  Port=4
  wires:
  I0_comp/1 -> 7/2, 6/2
  14/1 -> 6/1
  5/1 -> 7/1
  13/1 -> 14/2
  12/1 -> 5/2
  4/1 -> 14/1, 6/3
  3/1 -> 5/1, 7/3
  2/1 -> 3/2, 4/2, 12/2, 13/2
  I30_im/1 -> 13/1
  I30_re/1 -> 12/1
  11/1 -> 9/1, 8/1
  1/1 -> 11/2
  10/1 -> 11/1
  Fi_T/1 -> 10/2
  Fi_CT/1 -> 10/1
  8/1 -> orto_MUL_orto/4(F2im)
  9/1 -> orto_MUL_orto/3(F2re)
  7/1 -> orto_MUL_orto/1(F1re)
  6/1 -> orto_MUL_orto/2(F1im)
  orto_MUL_orto/2(Fim) -> I_im/1, module/2, orto_to_arg/2(im)
  orto_MUL_orto/1(Fre) -> I_re/1, module/1, orto_to_arg/1(re)
  module/1 -> I_eff/1
  orto_to_arg/1(arg) -> I_arg/1
  I_im_in/1 -> 4/1
  I_re_in/1 -> 3/1
  K_T/1 -> 2/2
  K_CT/1 -> 2/1

== system mylib/278_dzt_v1/diff_trans_calc_H2/Ia_diff_calc ==
  I_re_1 : Inport
  I_im_1 : Inport  Port=2
  I_re_2 : Inport  Port=3
  I_im_2 : Inport  Port=4
  fix : Inport  Port=5
  I_re_max_in : Inport  Port=6
  I_im_max_in : Inport  Port=7
  in_range_I : Inport  Port=8
  {1,3..6,12} (6 alike) : Switch  Criteria=u2 > Threshold
  10 : RelationalOperator  Operator=>  OutDataTypeStr=boolean  RndMeth=Simplest
  11 : Sum
  154 : Constant  Value=0
  2 : Sum
  module1 : Subsystem
  module2 : Subsystem
  I_re_diff : Outport
  I_im_diff1 : Outport  Port=2
  I_re_max : Outport  Port=3
  I_im_max : Outport  Port=4
  wires:
  fix/1 -> 4/2, 3/2
  I_re_2/1 -> 6/3
  I_im_2/1 -> 5/3
  I_im_max_in/1 -> module1/2(Im), 1/1
  I_re_max_in/1 -> 12/1, module1/1(Re)
  4/1 -> 2/2, 12/3, module2/1(Re)
  3/1 -> 1/3, 11/2, module2/2(Im)
  154/1 -> 5/1, 6/1, 4/3, 3/3
  in_range_I/1 -> 5/2, 6/2
  5/1 -> 3/1
  6/1 -> 4/1
  module2/1(Module) -> 10/2
  module1/1(Module) -> 10/1
  I_im_1/1 -> 11/1
  I_re_1/1 -> 2/1
  10/1 -> 1/2, 12/2
  2/1 -> I_re_diff/1
  11/1 -> I_im_diff1/1
  1/1 -> I_im_max/1
  12/1 -> I_re_max/1

== system mylib/278_dzt_v1/diff_trans_calc_H2/Ib_calc ==
  I_re_in : Inport
  I_im_in : Inport  Port=2
  I30_re : Inport  Port=3
  I30_im : Inport  Port=4
  K_CT : Inport  Port=5
  K_T : Inport  Port=6
  I0_comp : Inport  Port=7
  Fi_CT : Inport  Port=8
  Fi_T : Inport  Port=9
  1 : Constant  Value=0.017453292519
  10 : Sum  Inputs=+-
  {2..4,11..13} (6 alike) : Product
  14 : Sum  Inputs=+-
  5 : Sum  Inputs=+-
  6 : Switch  Criteria=u2 > Threshold
  7 : Switch  Criteria=u2 > Threshold
  8 : Trigonometry
  9 : Trigonometry  Operator=cos
  module : $bdroot/module  SystemSampleTime=-1  Latency=0  AutoFrameSizeCalculation=off
  orto_MUL_orto : Subsystem
  orto_to_arg : Subsystem
  I_re : Outport
  I_im : Outport  Port=2
  I_eff : Outport  Port=3
  I_arg : Outport  Port=4
  wires:
  I0_comp/1 -> 7/2, 6/2
  14/1 -> 6/1
  5/1 -> 7/1
  13/1 -> 14/2
  12/1 -> 5/2
  4/1 -> 14/1, 6/3
  3/1 -> 5/1, 7/3
  2/1 -> 3/2, 4/2, 12/2, 13/2
  I30_im/1 -> 13/1
  I30_re/1 -> 12/1
  11/1 -> 9/1, 8/1
  1/1 -> 11/2
  10/1 -> 11/1
  Fi_T/1 -> 10/2
  Fi_CT/1 -> 10/1
  8/1 -> orto_MUL_orto/4(F2im)
  9/1 -> orto_MUL_orto/3(F2re)
  7/1 -> orto_MUL_orto/1(F1re)
  6/1 -> orto_MUL_orto/2(F1im)
  orto_MUL_orto/2(Fim) -> I_im/1, module/2, orto_to_arg/2(im)
  orto_MUL_orto/1(Fre) -> I_re/1, module/1, orto_to_arg/1(re)
  module/1 -> I_eff/1
  orto_to_arg/1(arg) -> I_arg/1
  I_im_in/1 -> 4/1
  I_re_in/1 -> 3/1
  K_T/1 -> 2/2
  K_CT/1 -> 2/1

== system mylib/278_dzt_v1/diff_trans_calc_H2/Ib_diff_calc ==
  I_re_1 : Inport
  I_im_1 : Inport  Port=2
  I_re_2 : Inport  Port=3
  I_im_2 : Inport  Port=4
  fix : Inport  Port=5
  I_re_max_in : Inport  Port=6
  I_im_max_in : Inport  Port=7
  in_range_I : Inport  Port=8
  {1,3..6,12} (6 alike) : Switch  Criteria=u2 > Threshold
  10 : RelationalOperator  Operator=>  OutDataTypeStr=boolean  RndMeth=Simplest
  11 : Sum
  154 : Constant  Value=0
  2 : Sum
  module1 : Subsystem
  module2 : Subsystem
  I_re_diff : Outport
  I_im_diff1 : Outport  Port=2
  I_re_max : Outport  Port=3
  I_im_max : Outport  Port=4
  wires:
  fix/1 -> 4/2, 3/2
  I_re_2/1 -> 6/3
  I_im_2/1 -> 5/3
  I_im_max_in/1 -> module1/2(Im), 1/1
  I_re_max_in/1 -> 12/1, module1/1(Re)
  4/1 -> 2/2, 12/3, module2/1(Re)
  3/1 -> 1/3, 11/2, module2/2(Im)
  154/1 -> 5/1, 6/1, 4/3, 3/3
  in_range_I/1 -> 5/2, 6/2
  5/1 -> 3/1
  6/1 -> 4/1
  module2/1(Module) -> 10/2
  module1/1(Module) -> 10/1
  I_im_1/1 -> 11/1
  I_re_1/1 -> 2/1
  10/1 -> 1/2, 12/2
  2/1 -> I_re_diff/1
  11/1 -> I_im_diff1/1
  1/1 -> I_im_max/1
  12/1 -> I_re_max/1

== system mylib/278_dzt_v1/diff_trans_calc_H2/Ic_calc ==
  I_re_in : Inport
  I_im_in : Inport  Port=2
  I30_re : Inport  Port=3
  I30_im : Inport  Port=4
  K_CT : Inport  Port=5
  K_T : Inport  Port=6
  I0_comp : Inport  Port=7
  Fi_CT : Inport  Port=8
  Fi_T : Inport  Port=9
  1 : Constant  Value=0.017453292519
  10 : Sum  Inputs=+-
  {2..4,11..13} (6 alike) : Product
  14 : Sum  Inputs=+-
  5 : Sum  Inputs=+-
  6 : Switch  Criteria=u2 > Threshold
  7 : Switch  Criteria=u2 > Threshold
  8 : Trigonometry
  9 : Trigonometry  Operator=cos
  module : $bdroot/module  SystemSampleTime=-1  Latency=0  AutoFrameSizeCalculation=off
  orto_MUL_orto : Subsystem
  orto_to_arg : Subsystem
  I_re : Outport
  I_im : Outport  Port=2
  I_eff : Outport  Port=3
  I_arg : Outport  Port=4
  wires:
  I0_comp/1 -> 7/2, 6/2
  14/1 -> 6/1
  5/1 -> 7/1
  13/1 -> 14/2
  12/1 -> 5/2
  4/1 -> 14/1, 6/3
  3/1 -> 5/1, 7/3
  2/1 -> 3/2, 4/2, 12/2, 13/2
  I30_im/1 -> 13/1
  I30_re/1 -> 12/1
  11/1 -> 9/1, 8/1
  1/1 -> 11/2
  10/1 -> 11/1
  Fi_T/1 -> 10/2
  Fi_CT/1 -> 10/1
  8/1 -> orto_MUL_orto/4(F2im)
  9/1 -> orto_MUL_orto/3(F2re)
  7/1 -> orto_MUL_orto/1(F1re)
  6/1 -> orto_MUL_orto/2(F1im)
  orto_MUL_orto/2(Fim) -> I_im/1, module/2, orto_to_arg/2(im)
  orto_MUL_orto/1(Fre) -> I_re/1, module/1, orto_to_arg/1(re)
  module/1 -> I_eff/1
  orto_to_arg/1(arg) -> I_arg/1
  I_im_in/1 -> 4/1
  I_re_in/1 -> 3/1
  K_T/1 -> 2/2
  K_CT/1 -> 2/1

== system mylib/278_dzt_v1/diff_trans_calc_H2/Ic_diff_calc ==
  I_re_1 : Inport
  I_im_1 : Inport  Port=2
  I_re_2 : Inport  Port=3
  I_im_2 : Inport  Port=4
  fix : Inport  Port=5
  I_re_max_in : Inport  Port=6
  I_im_max_in : Inport  Port=7
  in_range_I : Inport  Port=8
  {1,3..6,12} (6 alike) : Switch  Criteria=u2 > Threshold
  10 : RelationalOperator  Operator=>  OutDataTypeStr=boolean  RndMeth=Simplest
  11 : Sum
  154 : Constant  Value=0
  2 : Sum
  module1 : Subsystem
  module2 : Subsystem
  I_re_diff : Outport
  I_im_diff1 : Outport  Port=2
  I_re_max : Outport  Port=3
  I_im_max : Outport  Port=4
  wires:
  fix/1 -> 4/2, 3/2
  I_re_2/1 -> 6/3
  I_im_2/1 -> 5/3
  I_im_max_in/1 -> module1/2(Im), 1/1
  I_re_max_in/1 -> 12/1, module1/1(Re)
  4/1 -> 2/2, 12/3, module2/1(Re)
  3/1 -> 1/3, 11/2, module2/2(Im)
  154/1 -> 5/1, 6/1, 4/3, 3/3
  in_range_I/1 -> 5/2, 6/2
  5/1 -> 3/1
  6/1 -> 4/1
  module2/1(Module) -> 10/2
  module1/1(Module) -> 10/1
  I_im_1/1 -> 11/1
  I_re_1/1 -> 2/1
  10/1 -> 1/2, 12/2
  2/1 -> I_re_diff/1
  11/1 -> I_im_diff1/1
  1/1 -> I_im_max/1
  12/1 -> I_re_max/1

== system mylib/278_dzt_v1/diff_trans_calc_H2/jmp_cnt18_ph ==
  cnt_jmp0_in : Inport
  cnt_jmp_in : Inport  Port=2
  Ia_zero_in : Inport  Port=3
  Ib_zero_in : Inport  Port=4
  Ic_zero_in : Inport  Port=5
  Iall_zero_in : Inport  Port=6
  in_range_Ia : Inport  Port=7
  in_range_Ib : Inport  Port=8
  in_range_Ic : Inport  Port=9
  jmp_Ia : Inport  Port=10
  jmp_Ib : Inport  Port=11
  jmp_Ic : Inport  Port=12
  fix : Inport  Port=13
  {1,3,5..7,10} (6 alike) : Logic  AllPortsSameDT=off  OutDataTypeStr=boolean
  11 : Logic  Operator=NOT  AllPortsSameDT=off  OutDataTypeStr=boolean
  12 : Logic  Operator=OR  AllPortsSameDT=off  OutDataTypeStr=boolean
  13 : Logic  Operator=OR  AllPortsSameDT=off  OutDataTypeStr=boolean
  14 : Logic  Operator=OR  AllPortsSameDT=off  OutDataTypeStr=boolean
  15 : Logic  Inputs=4  AllPortsSameDT=off  OutDataTypeStr=boolean
  16 : Switch  Criteria=u2 > Threshold
  17 : Switch  Criteria=u2 > Threshold
  18 : Sum
  19 : Constant
  2 : Logic  Operator=NOT  AllPortsSameDT=off  OutDataTypeStr=boolean
  20 : Sum
  21 : Constant
  4 : Logic  Operator=NOT  AllPortsSameDT=off  OutDataTypeStr=boolean
  8 : Logic  Operator=OR  Inputs=3  AllPortsSameDT=off  OutDataTypeStr=boolean
  9 : Logic  Operator=OR  Inputs=3  AllPortsSameDT=off  OutDataTypeStr=boolean
  R_TRIG : $bdroot/R_TRIG  SystemSampleTime=-1  Latency=0  AutoFrameSizeCalculation=off
  R_TRIG1 : $bdroot/R_TRIG  SystemSampleTime=-1  Latency=0  AutoFrameSizeCalculation=off
  R_TRIG2 : $bdroot/R_TRIG  SystemSampleTime=-1  Latency=0  AutoFrameSizeCalculation=off
  cnt_jmp0 : Outport
  cnt_jmp : Outport  Port=2
  Ia_zero : Outport  Port=3
  Ib_zero : Outport  Port=4
  Ic_zero : Outport  Port=5
  Iall_zero : Outport  Port=6
  wires:
  cnt_jmp0_in/1 -> 16/3, 20/1
  R_TRIG2/1 -> 9/3, 6/2
  fix/1 -> 10/2, 1/2, 3/2
  cnt_jmp_in/1 -> 17/3, 18/1
  9/1 -> 17/2
  20/1 -> 16/1
  21/1 -> 20/2
  19/1 -> 18/2
  18/1 -> 17/1
  17/1 -> cnt_jmp/1
  16/1 -> cnt_jmp0/1
  8/1 -> 16/2
  15/1 -> Iall_zero/1
  14/1 -> Ic_zero/1
  13/1 -> Ib_zero/1
  12/1 -> Ia_zero/1
  Ia_zero_in/1 -> 12/1
  Ib_zero_in/1 -> 13/1
  Ic_zero_in/1 -> 14/1
  Iall_zero_in/1 -> 15/1
  R_TRIG1/1 -> 9/2, 5/2
  R_TRIG/1 -> 9/1, 7/2
  6/1 -> 8/3
  7/1 -> 8/1
  5/1 -> 8/2
  10/1 -> 6/1, 15/4, 14/2
  1/1 -> 5/1, 15/3, 13/2
  3/1 -> 7/1, 15/2, 12/2
  in_range_Ia/1 -> 4/1
  4/1 -> 3/1
  in_range_Ib/1 -> 2/1
  2/1 -> 1/1
  in_range_Ic/1 -> 11/1
  11/1 -> 10/1
  jmp_Ib/1 -> R_TRIG1/1
  jmp_Ic/1 -> R_TRIG2/1
  jmp_Ia/1 -> R_TRIG/1

== system mylib/278_dzt_v1/diff_trans_calc_H2/simpcomp ==
  FAre : Inport
  FAim : Inport  Port=2
  FBre : Inport  Port=3
  FBim : Inport  Port=4
  FCre : Inport  Port=5
  FCim : Inport  Port=6
  1 : Constant  Value=-0.5
  {3..5,9..11,18..23} (12 alike) : Sum
  {2,12..16} (6 alike) : Product
  17 : Constant  Value=0.33333333333
  6 : Constant  Value=0.8660254037844386
  7 : Constant  Value=-0.8660254037844386
  orto_MUL_orto : Subsystem
  orto_MUL_orto1 : Subsystem
  orto_MUL_orto2 : Subsystem
  orto_MUL_orto3 : Subsystem
  F0re : Outport
  F0im : Outport  Port=2
  F1re : Outport  Port=3
  F1im : Outport  Port=4
  F2re : Outport  Port=5
  F2im : Outport  Port=6
  wires:
  1/1 -> orto_MUL_orto1/3(F2re), orto_MUL_orto/3(F2re), orto_MUL_orto2/3(F2re), orto_MUL_orto3/3(F2re)
  6/1 -> orto_MUL_orto2/4(F2im), orto_MUL_orto/4(F2im)
  7/1 -> orto_MUL_orto3/4(F2im), orto_MUL_orto1/4(F2im)
  15/1 -> F2im/1
  14/1 -> F2re/1
  16/1 -> F1im/1
  13/1 -> F1re/1
  2/1 -> F0re/1
  12/1 -> F0im/1
  5/1 -> 2/1
  3/1 -> 12/1
  4/1 -> 13/1
  11/1 -> 16/1
  9/1 -> 14/1
  10/1 -> 15/1
  20/1 -> 10/2
  23/1 -> 9/2
  21/1 -> 11/2
  22/1 -> 4/2
  18/1 -> 3/1
  19/1 -> 5/1
  FAim/1 -> 10/1, 3/2, 11/1
  FAre/1 -> 9/1, 5/2, 4/1
  orto_MUL_orto2/2(Fim) -> 20/2
  orto_MUL_orto1/2(Fim) -> 20/1
  orto_MUL_orto2/1(Fre) -> 23/2
  orto_MUL_orto1/1(Fre) -> 23/1
  orto_MUL_orto3/2(Fim) -> 21/2
  orto_MUL_orto/2(Fim) -> 21/1
  orto_MUL_orto3/1(Fre) -> 22/2
  orto_MUL_orto/1(Fre) -> 22/1
  FBre/1 -> orto_MUL_orto1/1(F1re), 19/1, orto_MUL_orto/1(F1re)
  FBim/1 -> orto_MUL_orto1/2(F1im), 18/1, orto_MUL_orto/2(F1im)
  FCim/1 -> 18/2, orto_MUL_orto2/2(F1im), orto_MUL_orto3/2(F1im)
  FCre/1 -> orto_MUL_orto3/1(F1re), 19/2, orto_MUL_orto2/1(F1re)
  17/1 -> 15/2, 14/2, 13/2, 12/2, 2/2, 16/2

== system mylib/Inverse time-delay/ANSI Inverse time-delay/Equation ANSI ==
  B : Inport
  I : Inport  Port=2
  Ip : Inport  Port=3
  A : Inport  Port=4
  C : Inport  Port=5
  D : Inport  Port=6
  Add : Sum  Inputs=+-
  Add1 : Sum
  Constant18 : Constant  Value=20
  Constant3 : Constant
  Divide : Product  Inputs=*/
  Divide1 : Product  Inputs=*/
  Divide3 : Product  Inputs=**
  Math Function : Math  Operator=pow  SaturateOnIntegerOverflow=on
  Relational Operator : RelationalOperator  OutDataTypeStr=boolean  RndMeth=Simplest
  Switch : Switch  Criteria=u2 > Threshold
  Zero_check : Subsystem
  Zero_check1 : Subsystem
  td : Outport
  wires:
  I/1 -> Divide/1
  B/1 -> Divide1/1
  D/1 -> Divide3/2
  Divide3/1 -> td/1
  Ip/1 -> Zero_check/1(in)
  Zero_check/1(out) -> Divide/2
  Add/1 -> Zero_check1/1(in)
  Zero_check1/1(out) -> Divide1/2
  Constant3/1 -> Add/2
  Divide1/1 -> Add1/1
  Add1/1 -> Divide3/1
  C/1 -> Add1/2
  Divide/1 -> Switch/3, Relational Operator/1
  Constant18/1 -> Switch/1, Relational Operator/2
  Relational Operator/1 -> Switch/2
  Switch/1 -> Math Function/1
  A/1 -> Math Function/2
  Math Function/1 -> Add/1

== system mylib/Inverse time-delay/ANSI Inverse time-delay/Сoefficient_1 ==
  A_in : Inport
  B_in : Inport  Port=2
  C_in : Inport  Port=3
  N : Inport  Port=4
  Constant1 : Constant  Value=0.17966
  Constant3 : Constant  Value=2.0938
  Constant6 : Constant  Value=8.9341
  Switch : Switch  Criteria=u2 > Threshold
  Switch1 : Switch  Criteria=u2 > Threshold
  Switch2 : Switch  Criteria=u2 > Threshold
  A_out : Outport
  B_out : Outport  Port=2
  C_out : Outport  Port=3
  wires:
  Switch1/1 -> B_out/1
  Constant3/1 -> Switch/1
  Constant6/1 -> Switch1/1
  Switch/1 -> A_out/1
  N/1 -> Switch2/2, Switch/2, Switch1/2
  A_in/1 -> Switch/3
  B_in/1 -> Switch1/3
  C_in/1 -> Switch2/3
  Constant1/1 -> Switch2/1
  Switch2/1 -> C_out/1

== system mylib/Inverse time-delay/ANSI Inverse time-delay/Сoefficient_2 ==
  A_in : Inport
  B_in : Inport  Port=2
  C_in : Inport  Port=3
  N : Inport  Port=4
  Constant1 : Constant  Value=0.03393
  Constant3 : Constant  Value=1.2969
  Constant6 : Constant  Value=0.2663
  Switch : Switch  Criteria=u2 > Threshold
  Switch1 : Switch  Criteria=u2 > Threshold
  Switch2 : Switch  Criteria=u2 > Threshold
  A_out : Outport
  B_out : Outport  Port=2
  C_out : Outport  Port=3
  wires:
  Switch1/1 -> B_out/1
  Constant3/1 -> Switch/1
  Constant6/1 -> Switch1/1
  Switch/1 -> A_out/1
  N/1 -> Switch2/2, Switch/2, Switch1/2
  A_in/1 -> Switch/3
  B_in/1 -> Switch1/3
  C_in/1 -> Switch2/3
  Constant1/1 -> Switch2/1
  Switch2/1 -> C_out/1

== system mylib/Inverse time-delay/ANSI Inverse time-delay/Сoefficient_3 ==
  A_in : Inport
  B_in : Inport  Port=2
  C_in : Inport  Port=3
  N : Inport  Port=4
  Constant1 : Constant  Value=2.18592
  Constant3 : Constant
  Constant6 : Constant  Value=5.6143
  Switch : Switch  Criteria=u2 > Threshold
  Switch1 : Switch  Criteria=u2 > Threshold
  Switch2 : Switch  Criteria=u2 > Threshold
  A_out : Outport
  B_out : Outport  Port=2
  C_out : Outport  Port=3
  wires:
  Switch1/1 -> B_out/1
  Constant3/1 -> Switch/1
  Constant6/1 -> Switch1/1
  Switch/1 -> A_out/1
  N/1 -> Switch2/2, Switch/2, Switch1/2
  A_in/1 -> Switch/3
  B_in/1 -> Switch1/3
  C_in/1 -> Switch2/3
  Constant1/1 -> Switch2/1
  Switch2/1 -> C_out/1

== system mylib/Inverse time-delay/ANSI Inverse time-delay/Сoefficient_4 ==
  A_in : Inport
  B_in : Inport  Port=2
  C_in : Inport  Port=3
  N : Inport  Port=4
  Constant1 : Constant  Value=0.0228
  Constant3 : Constant  Value=0.02
  Constant6 : Constant  Value=0.0103
  Switch : Switch  Criteria=u2 > Threshold
  Switch1 : Switch  Criteria=u2 > Threshold
  Switch2 : Switch  Criteria=u2 > Threshold
  A_out : Outport
  B_out : Outport  Port=2
  C_out : Outport  Port=3
  wires:
  Switch1/1 -> B_out/1
  Constant3/1 -> Switch/1
  Constant6/1 -> Switch1/1
  Switch/1 -> A_out/1
  N/1 -> Switch2/2, Switch/2, Switch1/2
  A_in/1 -> Switch/3
  B_in/1 -> Switch1/3
  C_in/1 -> Switch2/3
  Constant1/1 -> Switch2/1
  Switch2/1 -> C_out/1

== system mylib/Inverse time-delay/ANSI Inverse time-delay/Сoefficient_5 ==
  A_in : Inport
  B_in : Inport  Port=2
  C_in : Inport  Port=3
  N : Inport  Port=4
  Constant1 : Constant  Value=0.0982
  Constant3 : Constant  Value=2
  Constant6 : Constant  Value=3.922
  Switch : Switch  Criteria=u2 > Threshold
  Switch1 : Switch  Criteria=u2 > Threshold
  Switch2 : Switch  Criteria=u2 > Threshold
  A_out : Outport
  B_out : Outport  Port=2
  C_out : Outport  Port=3
  wires:
  Switch1/1 -> B_out/1
  Constant3/1 -> Switch/1
  Constant6/1 -> Switch1/1
  Switch/1 -> A_out/1
  N/1 -> Switch2/2, Switch/2, Switch1/2
  A_in/1 -> Switch/3
  B_in/1 -> Switch1/3
  C_in/1 -> Switch2/3
  Constant1/1 -> Switch2/1
  Switch2/1 -> C_out/1
